simulink model "GA_PID_Optimization"  (R2023b)
settings: Solver=VariableStepAuto  StartTime=0.0  StopTime=10  RelTol=1e-3
settings Model: Creator=movus  LastModifiedBy=movus

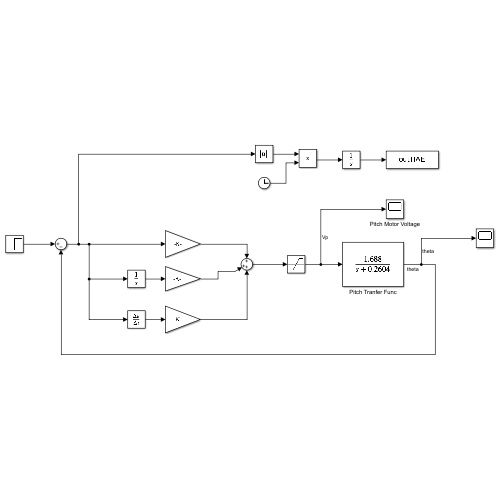
[thumbnail: Simulink's stored preview of the top-level diagram]
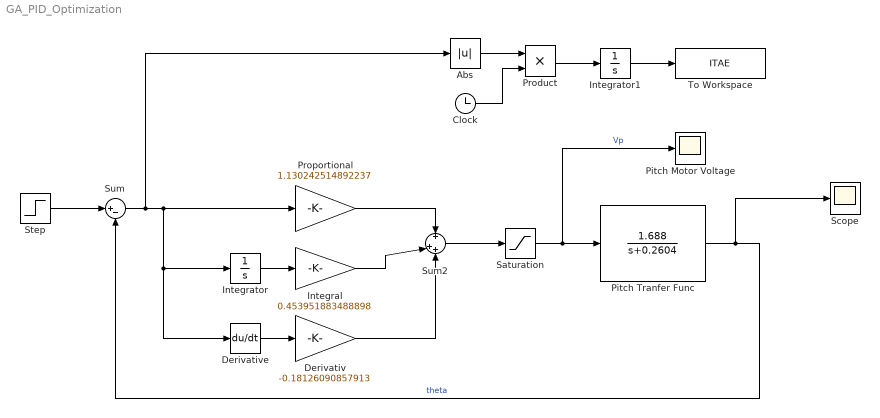
== system GA_PID_Optimization ==
  Abs : Abs  SaturateOnIntegerOverflow=off
  Clock : Clock
  Derivativ : Gain  Gain=-0.18126090857913
  Derivative : Derivative
  Integral : Gain  Gain=0.453951883488898
  Integrator : Integrator
  Integrator1 : Integrator
  Pitch Motor Voltage : Scope
  Pitch Tranfer Func : TransferFcn  Numerator=[1.688]  Denominator=[1 0.2604]
  Product : Product
  Proportional : Gain  Gain=1.130242514892237
  Saturation : Saturate  UpperLimit=12  LowerLimit=-12
  Scope : Scope
  Step : Step  Time=0  After=10  SampleTime=0
  Sum : Sum  Inputs=|+-
  Sum2 : Sum  Inputs=+|++
  To Workspace : ToWorkspace  VariableName=ITAE  SampleTime=-1
  wires:
  Step/1 -> Sum/1
  Integral/1 -> Sum2/2
  Derivativ/1 -> Sum2/3
  Integrator/1 -> Integral/1
  Sum/1 -> Abs/1, Integrator/1, Derivative/1, Proportional/1
  Sum2/1 -> Saturation/1
  Saturation/1 -> Pitch Tranfer Func/1, Pitch Motor Voltage/1  "Vp"
  Derivative/1 -> Derivativ/1
  Pitch Tranfer Func/1 -> Scope/1, Sum/2  "theta"
  Proportional/1 -> Sum2/1
  Abs/1 -> Product/1
  Clock/1 -> Product/2
  Product/1 -> Integrator1/1
  Integrator1/1 -> To Workspace/1
